simulink model "GalvoModel_servolike_v2_simpli"  (R2013a)
settings: Solver=ode45  StartTime=0.0  StopTime=10.0  RelTol=1e-3
values from neighbouring files (symbols this model uses):
  BEM = 108e-6    (= 0.000108)    [GalvoModel_thesis2_proc.m]
  CL = 180e-6    (= 0.00018)    [GalvoModel_thesis2_proc.m]    (also in GalvoModel_v4_sys.m = @(x,n) repmat(x, 1, n))
  CR = 2.79    [GalvoModel_thesis2_proc.m]
  FR = 4e-6    (= 4e-06)    [GalvoModel_thesis2_proc.m]
  KTR = 47e-3    (= 0.047)    [GalvoModel_thesis2_proc.m]
  RIN = 1.25e-8    (= 1.25e-08)    [GalvoModel_thesis2_proc.m]
  TRC = 6.17e-3    (= 0.00617)    [GalvoModel_thesis2_proc.m]
settings Model: Creator=mainster  LastModifiedBy=mainster
settings DebuggingCC: SolverPrmCheckMsg=none

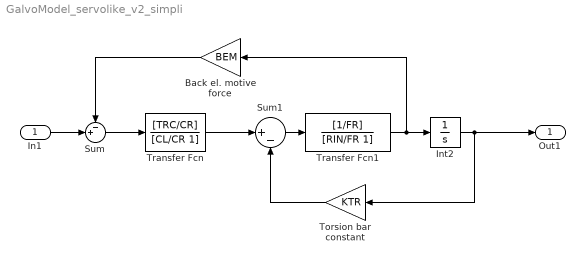
== system GalvoModel_servolike_v2_simpli ==
  In1 : Inport
  Back el. motive force : Gain  Gain=BEM
  Int2 : Integrator
  Sum : Sum  Inputs=-+|
  Sum1 : Sum  Inputs=|+-
  Torsion bar constant : Gain  Gain=KTR
  Transfer Fcn : TransferFcn  Numerator=[TRC/CR]  Denominator=[CL/CR 1]
  Transfer Fcn1 : TransferFcn  Numerator=[1/FR]  Denominator=[RIN/FR 1]
  Out1 : Outport
  wires:
  In1/1 -> Sum/2
  Sum/1 -> Transfer Fcn/1
  Transfer Fcn/1 -> Sum1/1
  Sum1/1 -> Transfer Fcn1/1
  Transfer Fcn1/1 -> Back el. motive force/1, Int2/1
  Torsion bar constant/1 -> Sum1/2
  Int2/1 -> Out1/1, Torsion bar constant/1
  Back el. motive force/1 -> Sum/1
